simulink model "MSD_Estimate"  (R2025b)
settings: Solver=FixedStepAuto  StartTime=0.0  StopTime=60  FixedStep=0.001  RelTol=1e-3
values from neighbouring files (symbols this model uses):
  b = 0.028    [KalmanFilter_model_MSD.m]    (also in MSD_Estimate_Parameter.m = 0.037)
  k = 29.839    [KalmanFilter_model_MSD.m]    (also in MSD_Estimate_Parameter.m)
  m = (0.039*Nut) + (0.145)    (= 0.34)    [KalmanFilter_model_MSD.m]    (also in MSD_Estimate_Parameter.m)
  x_inti = 0.0803448    [MSD_Estimate_Parameter.m]
settings Model: Creator=Akkarasaknarong  LastModifiedBy=Akkarasaknarong
settings DataIOCC: OutputOption=AdditionalOutputTimes  OutputTimes=SDO_OutputTimes  ReturnWorkspaceOutputsName=SDOSimTest_Log

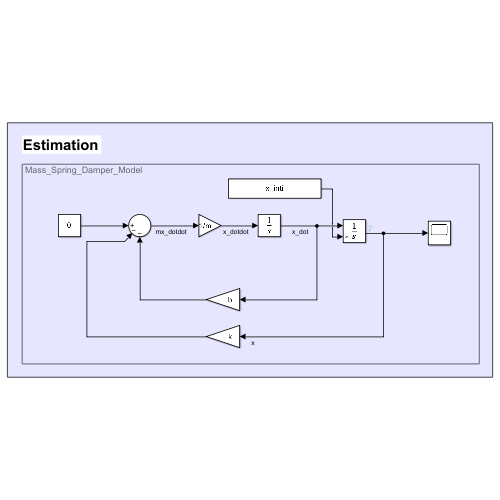
[thumbnail: Simulink's stored preview of the top-level diagram]
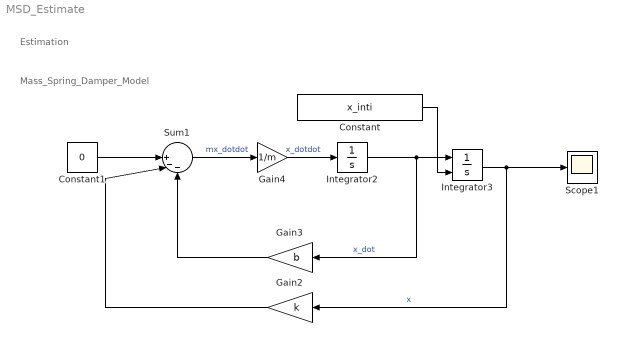
== system MSD_Estimate ==
  note: Mass_Spring_Damper_Model
  note: Estimation
  Constant : Constant  Value=x_inti
  Constant1 : Constant  Value=0
  Gain2 : Gain  Gain=k
  Gain3 : Gain  Gain=b
  Gain4 : Gain  Gain=1/m
  Integrator2 : Integrator
  Integrator3 : Integrator  InitialConditionSource=external
  Scope1 : Scope
  Sum1 : Sum  Inputs=||+--
  wires:
  Constant1/1 -> Sum1/1
  Gain4/1 -> Integrator2/1  "x_dotdot"
  Gain2/1 -> Sum1/2
  Sum1/1 -> Gain4/1  "mx_dotdot"
  Integrator3/1 -> Scope1/1, Gain2/1  "x"
  Integrator2/1 -> Gain3/1, Integrator3/1  "x_dot"
  Gain3/1 -> Sum1/3
  Constant/1 -> Integrator3/2
